simulink model "blockdiagram_2"  (R2021a)
settings: Solver=FixedStepDiscrete  StartTime=0.0  StopTime=135  FixedStep=0.001  RelTol=1e-3  EnableMultiTasking=on
PreLoadFcn:
  | set_param(gcs, 'RTWSystemTargetFile', 'franka_emika_panda.tlc');
  | initblockdiagram_1();
undefined symbols (not defined in the file or in its folder): amp, DiscIntNeverNeededParam, dof, init_delay
libraries: spsSampleandHoldLib x12, franka_simulink_library x4, simulink x1, etargetslib x1, dspnetwork x1
settings Model: ExtModeTrigDuration=10000  Creator=vasi_ko  LastModifiedBy=Bosma
settings SolverCC: AlgebraicLoopSolver=TrustRegion
settings DataIOCC: ExternalInput=identinput_2.getElement(1)  LimitDataPoints=on  SaveFormat=Array  ReturnWorkspaceOutputs=off
settings OptimizationCC: DefaultParameterBehavior=Inlined  EnhancedBackFolding=on  PassReuseOutputArgsThreshold=0  OptimizeBlockOrder=speed  DifferentSizesBufferReuse=on  OptimizationCustomize=off
settings DebuggingCC: SolverPrmCheckMsg=warning  ParameterTunabilityLossMsg=error  SFUnexpectedBacktrackingDiag=warning  SFNoUnconditionalDefaultTransitionDiag=warning  SFExecutionAtInitializationDiag=none  SFMachineParentedDataDiag=warning  ArithmeticOperatorsInVariantConditions=warning
settings HardwareCC: ProdBitPerLong=64  ProdHWDeviceType=Intel->x86-64 (Linux 64)
settings ModelReferenceCC: PropagateSignalLabelsOutOfModel=off
settings SFSimCC: SimUseLocalCustomCode=off  MATLABDynamicMemAlloc=off  CustomCodeUndefinedFunction=UseInterfaceOnly  SimTargetLang=C++
settings RTWCC: Description=Generic Real-Time Target  SystemTargetFile=franka_emika_panda.tlc  RTWVerbose=off  RTWUseLocalCustomCode=off  Toolchain=Franka Simulink | gmake (64-bit linux)  BuildConfiguration=Faster Runs  TargetLang=C++  DLArmComputeVersion=20.02.1
settings CodeAppCC: ForceParamTrailComments=on  OperatorAnnotations=on
settings STFCustomTargetCC: TargetLangStandard=C99 (ISO)  ModelReferenceCompliant=off  MATLABClassNameForMDSCustomization=Simulink.SoftwareTarget.TargetSpecificTriggerConfigurationBase  UseToolchainInfoCompliant=off  SystemTargetFile=franka_emika_panda.tlc
settings GRTTargetCC: ModelReferenceCompliant=off  ParMdlRefBuildCompliant=off  CompOptLevelCompliant=off  ConcurrentExecutionCompliant=off  CombineOutputUpdateFcns=off  MatFileLogging=off  MATLABClassNameForMDSCustomization=Simulink.SoftwareTarget.TargetSpecificTriggerConfigurationBase  CPPClassGenCompliant=off  GRTInterface=on  UseToolchainInfoCompliant=off
settings ConfigComp: CovMetricSettings=dw  CovSaveCumulativeToWorkspaceVar=on  CovSaveSingleToWorkspaceVar=on  CovExternalEMLEnable=off  CovSFcnEnable=off

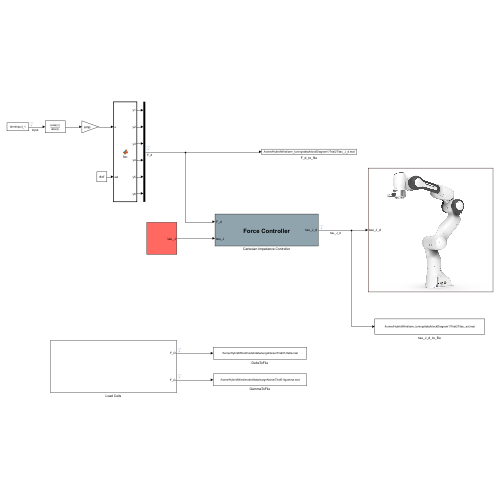
[thumbnail: Simulink's stored preview of the top-level diagram]
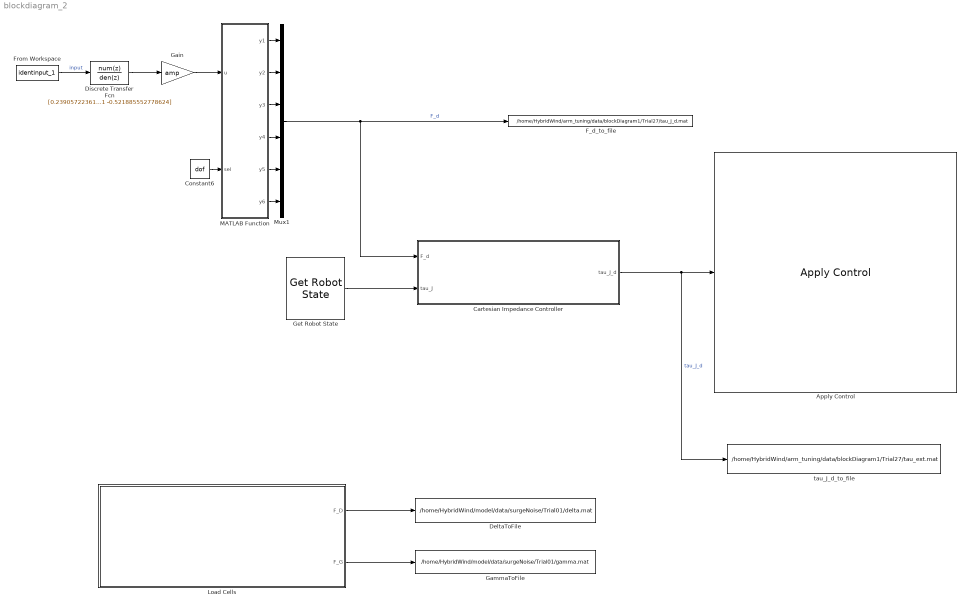
== system blockdiagram_2 ==
  Apply Control : franka_simulink_library/Apply Control  robot_ip=robot_ip  gripper_attached=off  control_mode=Torque Control  controller_choice=Joint Impedance Controller  elbow_control=on  collision_thresholds=100*ones(1,52)  joint_impedance=joint_impedance  cartesian_impedance=cartesian_impedance  load_inertia=load_inertia  EE_T_K=EE_T_K  init_joint_configuration_req=off  init_joint_configuration=[0.00392584915725334;-0.104076810189763;0.0404703493577216;-2.7334242600631;0.0113035300040543;2.63364770337236;0.372162046953987]
  Cartesian Impedance Controller : Subsystem
      mask Display:
      | disp('{\bf\fontsize{18}Force Controller}', 'texmode','on');
      | %
      | % block_icon('Controller')
      | %
      | port_label('input',1,'F_d');
      | port_label('input',2,'tau_J');
      | 
      | port_label('output',1,'tau_J_d');
  Constant6 : Constant  Value=dof
  DeltaToFile : ToFile  Filename=/home/HybridWind/model/data/surgeNoise/Trial01/delta.mat  MatrixName=delta
  Discrete Transfer Fcn : DiscreteTransferFcn  Numerator=[0.239057223610688 0.239057223610688]  Denominator=[1 -0.521885552778624]
  F_d_to_file : ToFile  Filename=/home/HybridWind/arm_tuning/data/blockDiagram1/Trial27/tau_J_d.mat  MatrixName=tau_J_d
  From Workspace : FromWorkspace  VariableName=identinput_1  SampleTime=0.001
  Gain : Gain  Gain=amp
  GammaToFile : ToFile  Filename=/home/HybridWind/model/data/surgeNoise/Trial01/gamma.mat  MatrixName=gamma
  Get Robot State : franka_simulink_library/Get Robot State  robot_ip=robot_ip  signals_requested='tau_J'
  Load Cells : Subsystem
  MATLAB Function : MATLAB Function  TreatAsAtomicUnit=on
  Mux1 : Mux  Inputs=6
  tau_J_d_to_file : ToFile  Filename=/home/HybridWind/arm_tuning/data/blockDiagram1/Trial27/tau_ext.mat  MatrixName=tau_ext
  wires:
  Get Robot State/1 -> Cartesian Impedance Controller/2(tau_J)
  Mux1/1 -> Cartesian Impedance Controller/1(F_d), F_d_to_file/1  "F_d"
  MATLAB Function/6(y6) -> Mux1/6
  Constant6/1 -> MATLAB Function/2(sel)
  MATLAB Function/5(y5) -> Mux1/5
  MATLAB Function/1(y1) -> Mux1/1
  MATLAB Function/2(y2) -> Mux1/2
  MATLAB Function/3(y3) -> Mux1/3
  MATLAB Function/4(y4) -> Mux1/4
  Gain/1 -> MATLAB Function/1(u)
  Discrete Transfer Fcn/1 -> Gain/1
  From Workspace/1 -> Discrete Transfer Fcn/1  "input"
  Cartesian Impedance Controller/1(tau_J_d) -> tau_J_d_to_file/1, Apply Control/1  "tau_J_d"
  Load Cells/1(F_D) -> DeltaToFile/1
  Load Cells/2(F_G) -> GammaToFile/1

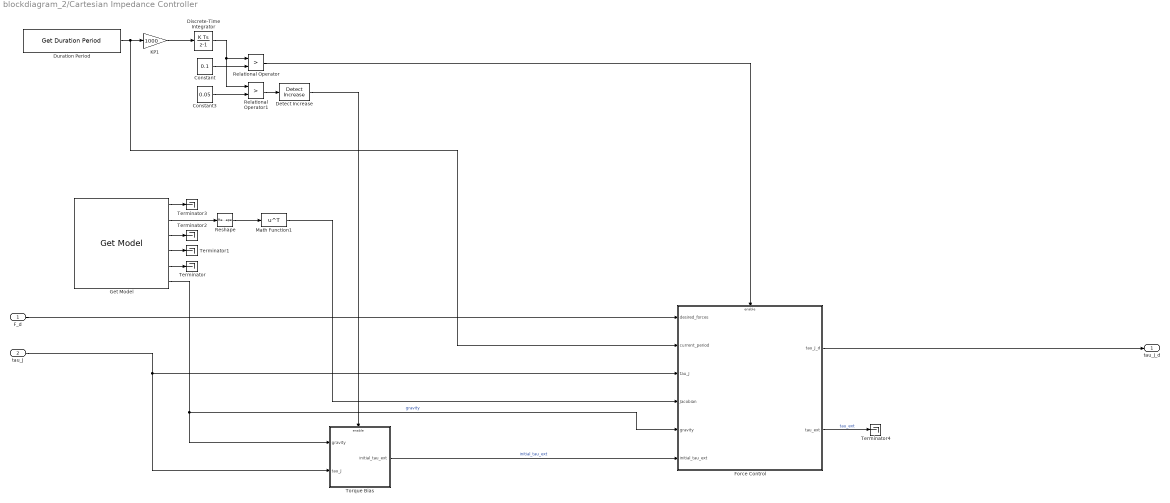
== system blockdiagram_2/Cartesian Impedance Controller ==
  F_d : Inport
  tau_J : Inport  Port=2
  Constant : Constant  Value=0.1
  Constant3 : Constant  Value=0.05
  Detect Increase : simulink/Logic and Bit Operations/Detect Increase  vinit=0.0  OutDataTypeStr=boolean
  Discrete-Time Integrator : DiscreteIntegrator  SampleTime=-1  ICPrevOutput=DiscIntNeverNeededParam  ICPrevScaledInput=DiscIntNeverNeededParam
  Duration Period : franka_simulink_library/Get Duration Period  robot_ip=robot_ip
  Force Control : Subsystem
  Get Model : franka_simulink_library/Get Model  robot_ip=robot_ip
  KP1 : Gain  Gain=1000
  Math Function1 : Math  Operator=transpose  SignedPower=on  SaturateOnIntegerOverflow=on
  Relational Operator : RelationalOperator  Operator=>  OutDataTypeStr=boolean  RndMeth=Nearest
  Relational Operator1 : RelationalOperator  Operator=>  OutDataTypeStr=boolean  RndMeth=Nearest
  Reshape : Reshape  OutputDimensionality=Customize  OutputDimensions=[6,7]
  Terminator{,1..4} (5 alike) : Terminator
  Torque Bias : Subsystem
  tau_J_d : Outport  VectorParamsAs1DForOutWhenUnconnected=off
  wires:
  Get Model/5 -> Terminator/1
  Get Model/4 -> Terminator1/1
  Get Model/2 -> Reshape/1
  tau_J/1 -> Force Control/3(tau_J), Torque Bias/2(tau_J)
  Discrete-Time Integrator/1 -> Relational Operator1/1, Relational Operator/1
  Constant/1 -> Relational Operator/2
  KP1/1 -> Discrete-Time Integrator/1
  Force Control/1(tau_J_d) -> tau_J_d/1
  Torque Bias/1(initial_tau_ext) -> Force Control/6(initial_tau_ext)  "initial_tau_ext"
  Get Model/6 -> Torque Bias/1(gravity), Force Control/5(gravity)  "gravity"
  Relational Operator/1 -> Force Control/Enable
  Reshape/1 -> Math Function1/1
  Duration Period/1 -> KP1/1, Force Control/2(current_period)
  Constant3/1 -> Relational Operator1/2
  Relational Operator1/1 -> Detect Increase/1
  Detect Increase/1 -> Torque Bias/Enable
  Force Control/2(tau_ext) -> Terminator4/1  "tau_ext"
  Get Model/1 -> Terminator3/1
  Math Function1/1 -> Force Control/4(Jacobian)
  Get Model/3 -> Terminator2/1
  F_d/1 -> Force Control/1(desired_forces)

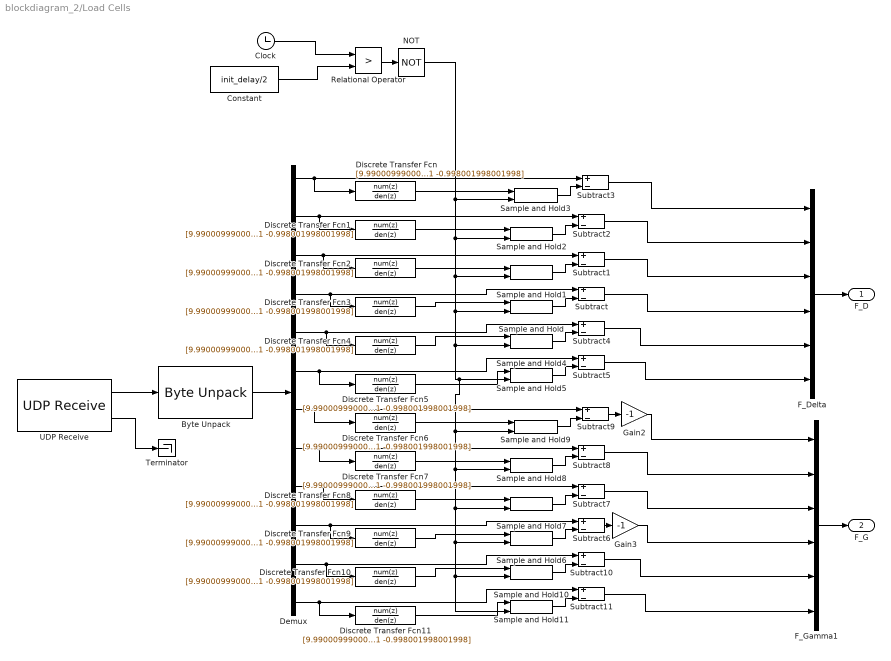
== system blockdiagram_2/Load Cells ==
  Byte Unpack : etargetslib/Byte Unpack  dimensions={[12]}  datatypes={'double'}  byteAlign=1
  Clock : Clock
  Constant : Constant  Value=init_delay/2
  Demux : Demux  Outputs=12
  Discrete Transfer Fcn{,1..11} (12 alike) : DiscreteTransferFcn  Numerator=[9.990009990009990e-04 9.990009990009990e-04]  Denominator=[1 -0.998001998001998]
  F_Delta : Mux  Inputs=6
  F_Gamma1 : Mux  Inputs=6
  Gain2 : Gain  Gain=-1
  Gain3 : Gain  Gain=-1
  NOT : Logic  Operator=NOT  IconShape=distinctive  AllPortsSameDT=off  OutDataTypeStr=boolean
  Relational Operator : RelationalOperator  Operator=>  OutDataTypeStr=boolean  RndMeth=Simplest
  Sample and Hold{,1..11} (12 alike) : spsSampleandHoldLib/Sample and Hold  ic=0  Ts=0
  Subtract{,1..11} (12 alike) : Sum  Inputs=+-
  Terminator : Terminator
  UDP Receive : dspnetwork/UDP Receive  localURL='0.0.0.0'  localPort=8002  remoteURL='10.10.10.15'  remotePort=-1  recvBufferSize=8192  dims=96  signalDatatype=uint8  isComplex=off  isVarSize=off  showBlockingTime=on  blockingTime=inf  sampletime=0.001  blockPlatform=HOST
  F_D : Outport
  F_G : Outport  Port=2
  wires:
  UDP Receive/1 -> Byte Unpack/1
  Constant/1 -> Relational Operator/2
  Relational Operator/1 -> NOT/1
  Sample and Hold/1 -> Subtract/2
  UDP Receive/2 -> Terminator/1
  Demux/4 -> Discrete Transfer Fcn3/1, Subtract/1
  Clock/1 -> Relational Operator/1
  Byte Unpack/1 -> Demux/1
  Demux/3 -> Discrete Transfer Fcn2/1, Subtract1/1
  Sample and Hold1/1 -> Subtract1/2
  Subtract1/1 -> F_Delta/3
  Subtract2/1 -> F_Delta/2
  Sample and Hold2/1 -> Subtract2/2
  Demux/2 -> Discrete Transfer Fcn1/1, Subtract2/1
  Sample and Hold3/1 -> Subtract3/2
  Subtract4/1 -> F_Delta/5
  Sample and Hold4/1 -> Subtract4/2
  Demux/5 -> Discrete Transfer Fcn4/1, Subtract4/1
  Demux/6 -> Discrete Transfer Fcn5/1, Subtract5/1
  Sample and Hold5/1 -> Subtract5/2
  Subtract5/1 -> F_Delta/6
  Subtract3/1 -> F_Delta/1
  Subtract/1 -> F_Delta/4
  F_Delta/1 -> F_D/1
  Demux/1 -> Discrete Transfer Fcn/1, Subtract3/1
  Discrete Transfer Fcn/1 -> Sample and Hold3/1
  Discrete Transfer Fcn1/1 -> Sample and Hold2/1
  Discrete Transfer Fcn2/1 -> Sample and Hold1/1
  Discrete Transfer Fcn3/1 -> Sample and Hold/1
  Discrete Transfer Fcn4/1 -> Sample and Hold4/1
  Discrete Transfer Fcn5/1 -> Sample and Hold5/1
  Discrete Transfer Fcn11/1 -> Sample and Hold11/1
  Discrete Transfer Fcn10/1 -> Sample and Hold10/1
  Discrete Transfer Fcn9/1 -> Sample and Hold6/1
  Discrete Transfer Fcn8/1 -> Sample and Hold7/1
  Discrete Transfer Fcn7/1 -> Sample and Hold8/1
  Discrete Transfer Fcn6/1 -> Sample and Hold9/1
  Demux/7 -> Subtract9/1, Discrete Transfer Fcn6/1
  F_Gamma1/1 -> F_G/1
  Gain3/1 -> F_Gamma1/4
  Gain2/1 -> F_Gamma1/1
  Subtract11/1 -> F_Gamma1/6
  Sample and Hold11/1 -> Subtract11/2
  NOT/1 -> Sample and Hold3/2, Sample and Hold2/2, Sample and Hold1/2, Sample and Hold6/2, Sample and Hold10/2, Sample and Hold11/2, Sample and Hold7/2, Sample and Hold8/2, Sample and Hold9/2, Sample and Hold5/2, Sample and Hold4/2, Sample and Hold/2
  Demux/12 -> Subtract11/1, Discrete Transfer Fcn11/1
  Demux/11 -> Subtract10/1, Discrete Transfer Fcn10/1
  Sample and Hold10/1 -> Subtract10/2
  Subtract10/1 -> F_Gamma1/5
  Subtract9/1 -> Gain2/1
  Sample and Hold9/1 -> Subtract9/2
  Demux/8 -> Subtract8/1, Discrete Transfer Fcn7/1
  Sample and Hold8/1 -> Subtract8/2
  Subtract8/1 -> F_Gamma1/2
  Subtract7/1 -> F_Gamma1/3
  Sample and Hold7/1 -> Subtract7/2
  Demux/9 -> Subtract7/1, Discrete Transfer Fcn8/1
  Demux/10 -> Subtract6/1, Discrete Transfer Fcn9/1
  Sample and Hold6/1 -> Subtract6/2
  Subtract6/1 -> Gain3/1

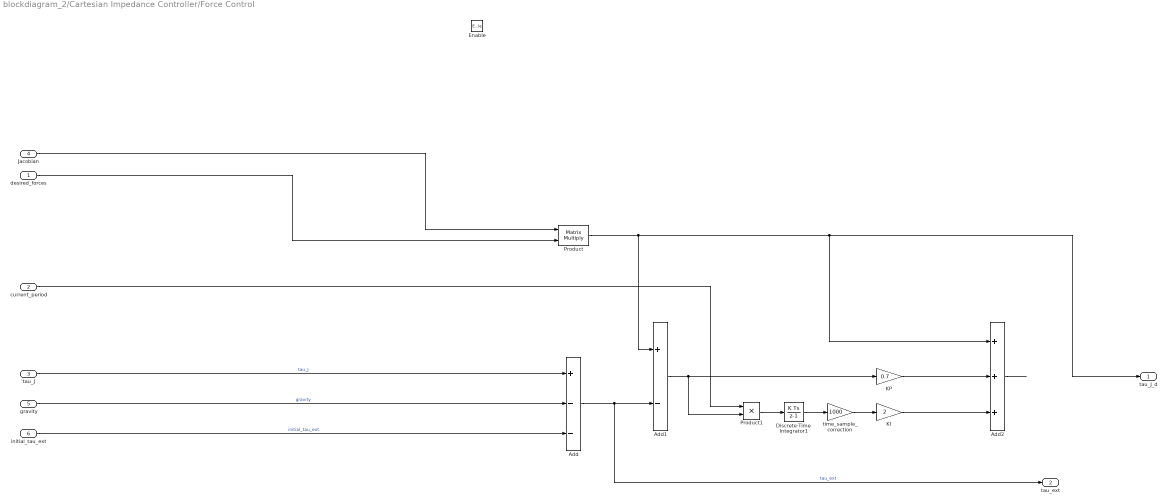
== system blockdiagram_2/Cartesian Impedance Controller/Force Control ==
  desired_forces : Inport
  current_period : Inport  Port=2
  tau_J : Inport  Port=3
  Jacobian : Inport  Port=4
  gravity : Inport  Port=5
  initial_tau_ext : Inport  Port=6
  Enable : EnablePort
  Add : Sum  Inputs=+--
  Add1 : Sum  Inputs=+-
  Add2 : Sum  Inputs=+++
  Discrete-Time Integrator1 : DiscreteIntegrator  SampleTime=0.001  ICPrevOutput=DiscIntNeverNeededParam  ICPrevScaledInput=DiscIntNeverNeededParam
  KI : Gain  Gain=2
  KP : Gain  Gain=0.7
  Product : Product  Multiplication=Matrix(*)
  Product1 : Product
  time_sample_correction : Gain  Gain=1000
  tau_J_d : Outport  InitialOutput=[0 0 0 0 0 0 0]  VectorParamsAs1DForOutWhenUnconnected=off
  tau_ext : Outport  Port=2  InitialOutput=[0 0 0 0 0 0 0]  VectorParamsAs1DForOutWhenUnconnected=off
  wires:
  Jacobian/1 -> Product/1
  tau_J/1 -> Add/1  "tau_J"
  gravity/1 -> Add/2  "gravity"
  Add/1 -> tau_ext/1, Add1/2  "tau_ext"
  Add1/1 -> Product1/2, KP/1
  Add2/1 -> ?
  Product1/1 -> Discrete-Time Integrator1/1
  current_period/1 -> Product1/1
  KI/1 -> Add2/3
  initial_tau_ext/1 -> Add/3  "initial_tau_ext"
  Product/1 -> Add1/1, tau_J_d/1, Add2/1
  KP/1 -> Add2/2
  desired_forces/1 -> Product/2
  Discrete-Time Integrator1/1 -> time_sample_correction/1
  time_sample_correction/1 -> KI/1

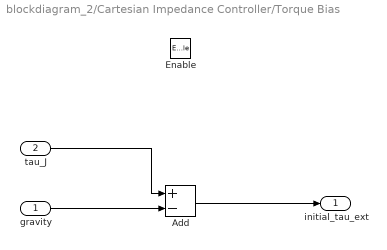
== system blockdiagram_2/Cartesian Impedance Controller/Torque Bias ==
  gravity : Inport
  tau_J : Inport  Port=2
  Enable : EnablePort
  Add : Sum  Inputs=+-
  initial_tau_ext : Outport  InitialOutput=[0 0 0 0 0 0 0]  VectorParamsAs1DForOutWhenUnconnected=off
  wires:
  tau_J/1 -> Add/1
  gravity/1 -> Add/2
  Add/1 -> initial_tau_ext/1

== matlab function blockdiagram_2/MATLAB Function ==
  data: u input; y1 output; sel input; y2 output; y3 output; y4 output; y5 output; y6 output
function [y1, y2, y3, y4, y5, y6] = fcn(u, sel)

y1 = 0;
y2 = 0;
y3 = 0;
y4 = 0;
y5 = 0;
y6 = 0;

switch sel
    case 1
        y1 = u;
    case 2
        y2 = u;
    case 3
        y3 = u;
    case 4
        y4 = u;
    case 5
        y5 = u;
    case 6
        y6 = u;
    otherwise
        y1 = 0;
end
